simulink model "HW11"  (Simulink 7.9)
settings: Solver=ode45  StartTime=0.0  StopTime=10.0  RelTol=1e-3
settings Model: Creator=alex  LastModifiedBy=alex

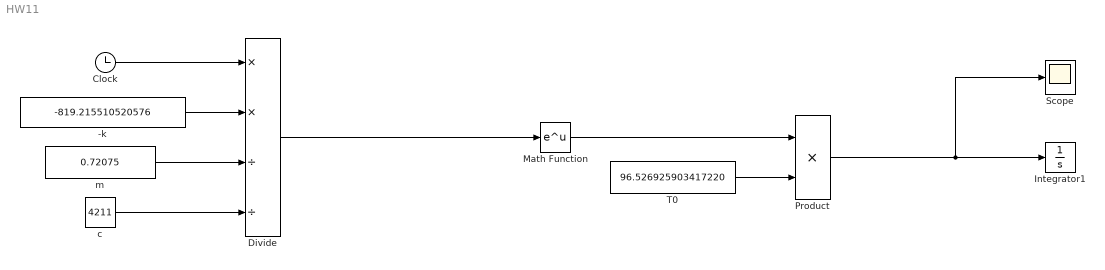
== system HW11 ==
  -k : Constant  Value=-819.215510520576
  Clock : Clock
  Divide : Product  Inputs=**//
  Integrator1 : Integrator  InitialCondition=100
  Math Function : Math  SaturateOnIntegerOverflow=on
  Product : Product  RndMeth=Zero
  Scope : Scope
  T0 : Constant  Value=96.526925903417220
  c : Constant  Value=4211
  m : Constant  Value=0.72075
  wires:
  Clock/1 -> Divide/1
  -k/1 -> Divide/2
  m/1 -> Divide/3
  c/1 -> Divide/4
  Divide/1 -> Math Function/1
  Math Function/1 -> Product/1
  Product/1 -> Integrator1/1, Scope/1
  T0/1 -> Product/2
